simulink model "Foc"  (R2020b)
settings: Solver=FixedStepAuto  StartTime=0.0  StopTime=2  FixedStep=0.000001  RelTol=1e-3
libraries: powerlib x6, pid_lib x3, simulink x1
settings Model: Creator=Anson  LastModifiedBy=Anson

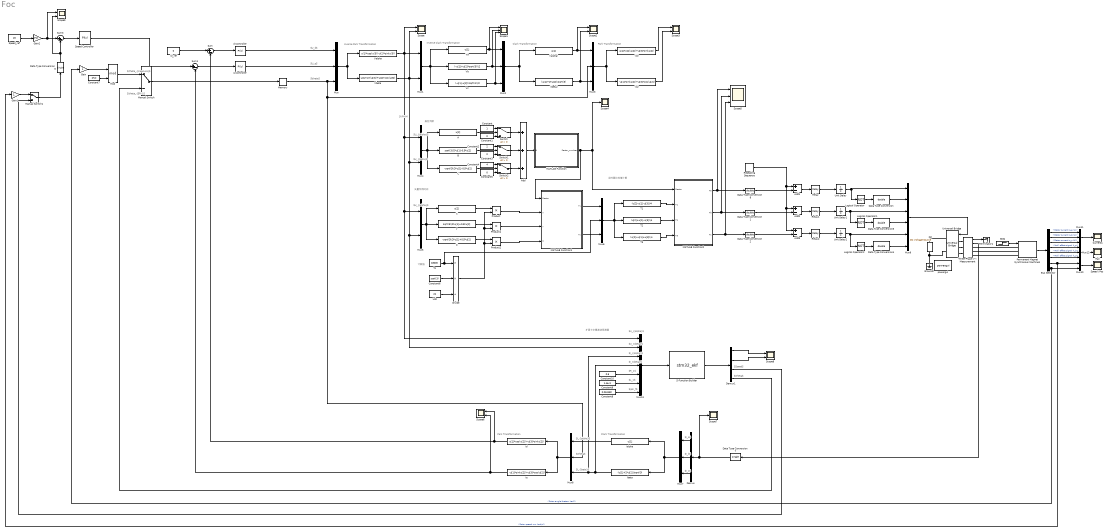
== system Foc ==
  note: $\theta$
  note: $U_q$
  note: $\theta$
  note: $\theta$
  note: $\theta_{EFK}$
  note: 扩展卡尔曼滤波观测器
  note: $I_a$
  note: $U_{\alpha}$
  note: 定时器比较值计算
  note: 矢量作用时间
  note: SVPWM
  note: 计数值
  note: Park Transformation
  note: Clark Transformation
  note: Inverse Clark Transformation
  note: Inverse Park Transformation
  note: 扇区判断
  note: Park Transformation
  note: Clark Transformation
  note: $U_{\beta}$
  note: $U_{\alpha}$
  note: $U_{\beta}$
  note: $I_b$
  note: $I_c$
  note: $U_{\alpha}$
  note: $I_{\alpha}$
  note: $I_{\beta}$
  note: $\psi_f$
  note: $L_s$
  note: $R_s$
  note: $\theta_{measure}$
  note: $U_d$
  note: $I_{\alpha}$
  note: $I_{\beta}$
  note: $Speed$
  (Ialpha) : Fcn  Expr=u[1]
  (Ibeta) : Fcn  Expr=(u[1]+2*u[2])/sqrt(3)
  (Id) : Fcn  Expr=u[1]*cos(u[2])+u[3]*sin(u[2])
  (Iq) : Fcn  Expr=-u[1]*sin(u[2])+u[3]*cos(u[2])
  A : Fcn  Expr=u[2]
  Add : Sum  Inputs=+++
  Add1 : Sum  Inputs=+-
  Add2 : Sum  Inputs=+-
  Add3 : Sum  Inputs=+-
  B : Fcn  Expr=sqrt(3)/2*u[1]-0.5*u[2]
  Bus Selector : BusSelector  OutputSignals=Stator current is_a (A),Stator current is_b (A),Stator current is_c (A),Hall effect signal h_a,Hall effect signal h_b,Hall effect signal h_c,Rotor speed wm (rad/s),Rotor angle thetam (rad)
  C : Fcn  Expr=-sqrt(3)/2*u[1]-0.5*u[2]
  Constant : Constant
  Constant1 : Constant  Value=0
  Constant10 : Constant  Value=0.6  OutDataTypeStr=single
  Constant2 : Constant  Value=2
  Constant3 : Constant  Value=0
  Constant4 : Constant  Value=4
  Constant5 : Constant  Value=0
  Constant6 : Constant  Value=sqrt(3)  OutDataTypeStr=single
  Constant7 : Constant  Value=2*pi  OutDataTypeStr=single
  Constant8 : Constant  Value=0.034182  OutDataTypeStr=single
  Constant9 : Constant  Value=1.4e-3  OutDataTypeStr=single
  Currents : Scope
  "DC " : powerlib/Electrical Sources/DC Voltage Source  Amplitude=24  Measurements=None
  Data Type Conversion{,1..4,8} (6 alike) : DataTypeConversion  OutDataTypeStr=double
  Data Type Conversion6 : DataTypeConversion  OutDataTypeStr=single
  Data Type Conversion7 : DataTypeConversion  OutDataTypeStr=single
  Demux : Demux  Outputs=3
  Demux1 : Demux
  Divide : Product  Inputs=**/
  Gain : Gain  OutDataTypeStr=single
  Gain1 : Gain  OutDataTypeStr=double
  Gain2 : Gain  Gain=2*pi  OutDataTypeStr=single
  Ground2 : powerlib/Elements/Ground  LConnTagsString=a
  Hall : Scope
  Ialpha : Fcn  Expr=u[1]
  Ibeta : Fcn  Expr=(u[1]+2*u[2])/sqrt(3)
  Id : Fcn  Expr=u[1]*cos(u[2])+u[3]*sin(u[2])
  Id_ref : Constant  Value=0  OutDataTypeStr=single
  Iq : Fcn  Expr=-u[1]*sin(u[2])+u[3]*cos(u[2])
  Logical Operator : Logic  Operator=NOT  AllPortsSameDT=off  OutDataTypeStr=boolean
  Logical Operator1 : Logic  Operator=NOT  AllPortsSameDT=off  OutDataTypeStr=boolean
  Logical Operator2 : Logic  Operator=NOT  AllPortsSameDT=off  OutDataTypeStr=boolean
  MATLAB Function : MATLAB Function  TreatAsAtomicUnit=on
  MATLAB Function1 : MATLAB Function  TreatAsAtomicUnit=on
  MATLAB Function2 : MATLAB Function  TreatAsAtomicUnit=on
  Manual Switch : ManualSwitch
  Manual Switch1 : ManualSwitch
  Memory : Memory
  Mod : Math  Operator=mod  SaturateOnIntegerOverflow=on
  Mux{,2..3,6..8,11..12} (8 alike) : Mux  Inputs=3
  Mux{1,4..5,10} (4 alike) : Mux  Inputs=2
  Mux13 : Mux  Inputs=7
  Mux9 : Mux  Inputs=6
  Permanent Magnet Synchronous Machine1 : powerlib/Machines/Permanent Magnet Synchronous Machine  NbPhases=3  FluxDistribution=Sinusoidal  RotorType=Round  MechanicalLoad=Torque Tm  PresetModel=No  ShowDetailedParameters=on  MeasurementBus=off  Resistance=0.6  Inductance=8.5e-3  dqInductances=[8.5e-3, 8.5e-3]  La=1.4e-3  MachineConstant=Flux linkage established by magnets (V.s)  Flux=0.034182  VoltageCst=6.1999  TorqueCst=0.051273  Flat=120  Mechanical=[1.1e-5,1e-4,1,0.02]  PolePairs=4  InitialConditions=[0,0, 0,0]  InitialConditions5ph=[0 0 0 0 0 0]  RefAngle=Aligned with phase A axis (original Park)  IterativeDiscreteModel=Trapezoidal non iterative  TsBlock=-1  TsPowergui=0
  Product : Product
  Product1 : Product
  Product2 : Product
  Relay : Relay  OffSwitchValue=-eps
  Relay1 : Relay  OffSwitchValue=-eps
  Relay2 : Relay  OffSwitchValue=-eps
  Repeating Sequence : simulink/Sources/Repeating Sequence  rep_seq_t=[0 0.0001 0.0002]  rep_seq_y=[0 9000 0]
  S-Function Builder : S-Function  InitFcn=try, set_param(gcb,'FunctionName','stm32_ekf'), end  FunctionName=stm32_ekf  SFunctionModules=stm32_ekf_wrapper  SFunctionDeploymentMode=off  EnableBusSupport=off  mask(S-Function Builder){}
      mask help: Simulink:masks:SFunctionBuilder_MD
      mask init:
      | val = [[.9  0.75 0.75 1 1 .9 .9 1]',[1 1 0.75 0.75 .9 .9 1 .9]'];try , sys = get_param(gcb,'SfunBuilderFcnName');if isempty(sys), sys = get_param(gcb,'FunctionName'); end,catch, sys = get_param(gcb,'FunctionName'); end
      settings: CopyFcn=set_param(gcbh,'LinkStatus','none')  PreSaveFcn=try, set_param(gcb,'FunctionName','stm32_ekf'), end  OpenFcn=sfunctionwizard(gcbh)
      mask Display: plot(val(:,1),val(:,2)),disp(sys),port_label('input',1,'u'),port_label('output',1,'y')
  Scope{,2..3,6,8..9} (6 alike) : Scope  NumInputPorts=2
  Scope1 : Scope  NumInputPorts=3
  Scope4 : Scope
  Scope5 : Scope  NumInputPorts=3
  Scope7 : Scope
  Speed / Pos : Scope
  Speed Controller : pid_lib/PID Controller  Controller=PI  Form=Ideal  TimeDomain=Discrete-time  UseExternalTs=off  SampleTime=-1  IntegratorMethod=Forward Euler  FilterMethod=Forward Euler  ControllerParametersSource=internal  P=0.005  I=6.0  D=0.0005  UseFilter=on  N=100  TunerSelectOption=Transfer Function Based (PID Tuner App)  InitialConditionSource=internal  InitialConditionForIntegrator=0  InitialConditionForFilter=0  DifferentiatorICPrevScaledInput=0  ExternalReset=none  TrackingMode=off  Kt=1  LimitOutput=on  SatLimitsSource=internal  UpperSaturationLimit=5.0  LowerSaturationLimit=-5.0  LinearizeAsGain=off  AntiWindupMode=back-calculation  Kb=0.015  PGainOutDataTypeStr=single  PProdOutDataTypeStr=single  POutMin=[]  POutMax=[]  IGainOutDataTypeStr=single  IProdOutDataTypeStr=single  IOutMin=[]  IOutMax=[]  DOutMin=[]  DOutMax=[]  NOutMin=[]  NOutMax=[]  SumOutDataTypeStr=single  SumOutMin=[]  SumOutMax=[]  SaturationOutDataTypeStr=single  SaturationOutMin=[]  SaturationOutMax=[]  PParamDataTypeStr=single  PParamMin=[]  PParamMax=[]  IParamDataTypeStr=single  IParamMin=[]  IParamMax=[]  DParamMin=[]  DParamMax=[]  NParamMin=[]  NParamMax=[]  KbParamDataTypeStr=single  KbParamMin=[]  KbParamMax=[]  KtParamMin=[]  KtParamMax=[]  KbOutDataTypeStr=single  KbOutMin=[]  KbOutMax=[]  KtOutMin=[]  KtOutMax=[]  IntegratorOutDataTypeStr=single  IntegratorOutMin=[]  IntegratorOutMax=[]  FilterOutMin=[]  FilterOutMax=[]  SumI1OutDataTypeStr=single  SumI1OutMin=[]  SumI1OutMax=[]  SumI2OutDataTypeStr=single  SumI2OutMin=[]  SumI2OutMax=[]  SumI3OutMin=[]  SumI3OutMax=[]  SumI4OutMin=[]  SumI4OutMax=[]  SumDOutMin=[]  SumDOutMax=[]  SumAccumDataTypeStr=single  SumI1AccumDataTypeStr=single  SumI2AccumDataTypeStr=single  DifferentiatorOutMin=[]  DifferentiatorOutMax=[]  FilterDiffOutCoefMin=[]  FilterDiffOutCoefMax=[]  ReciprocalOutMin=[]  ReciprocalOutMax=[]  SumDenOutMin=[]  SumDenOutMax=[]  SumNumOutMin=[]  SumNumOutMax=[]  DivideOutMin=[]  DivideOutMax=[]  UdiffTsProdOutMin=[]  UdiffTsProdOutMax=[]  NTsProdOutMin=[]  NTsProdOutMax=[]  UintegralTsProdOutMin=[]  UintegralTsProdOutMax=[]  UngainTsProdOutMin=[]  UngainTsProdOutMax=[]  IntegratorContinuousStateAttributes=''  IntegratorStateIdentifier=si  IntegratorStateMustResolveToSignalObject=off  IntegratorRTWStateStorageClass=Auto  FilterContinuousStateAttributes=''  FilterStateMustResolveToSignalObject=off  FilterRTWStateStorageClass=Auto  ParallelPVariant=Passthrough  IdealPVariant=InternalParameters  IVariant=InternalParameters  DVariant=Disabled  IntegratorVariant=Discrete  SatVariant=Enabled  AWVariant=BackCalculation  PCopyVariant=Disabled  TRVariant=Disabled  FdbkBlocksVariant=Forward  IdealPFdbkVariant=Disabled  SatFdbkVariant=Disabled  DerivativeFilterVariant=Disabled  NVariant=Disabled  NCopyVariant=Disabled_SignalSpec  FilterICVariant=Disabled  IntegratorICVariant=InternalICs  ExternalResetVariant=Disabled  TRSumVariant=Passthrough  SumFdbkVariant=Disabled  SumVariant=Sum_PI  TsampFilterVariant=InternalTs  TsampNgainVariant=Passthrough  TsampIntegralVariant=Passthrough  ExternalSaturationOutDataTypeStr=Inherit: Same as second input
  Speed_ref : Constant  Value=20  OutDataTypeStr=single
  Step : Step  Time=0  After=0  SampleTime=0
  Sum : Sum  Inputs=|+-
  Sum1 : Sum  Inputs=|+-
  Sum3 : Sum  Inputs=|+-  InputSameDT=on
  Switch : Switch  Criteria=u2 > Threshold
  Switch1 : Switch  Criteria=u2 > Threshold
  Switch2 : Switch  Criteria=u2 > Threshold
  T1 : Fcn  Expr=(u[2]-u[1]-u[3])/4
  T2 : Fcn  Expr=(u[2]+u[1]-u[3])/4
  T3 : Fcn  Expr=(u[2]+u[1]+u[3])/4
  Terminator1 : Terminator
  Three-Phase V-I Measurement : powerlib/Measurements/Three-Phase V-I Measurement  VoltageMeasurement=phase-to-ground  SetLabelV=off  LabelV=Vabc  Vpu=off  VpuLL=off  CurrentMeasurement=yes  SetLabelI=off  LabelI=Iabc  Ipu=off  Pbase=100e6  Vbase=500e3  OutputType=Complex  PhasorSimulation=off  PSBequivalent=0
  Ts : Constant  Value=18000  OutDataTypeStr=single
  Udc : Constant  Value=24  OutDataTypeStr=single
  Unit Delay : UnitDelay  SampleTime=-1  HasFrameUpgradeWarning=on
  Unit Delay1 : UnitDelay  SampleTime=-1  HasFrameUpgradeWarning=on
  Unit Delay2 : UnitDelay  SampleTime=-1  HasFrameUpgradeWarning=on
  Universal Bridge : powerlib/Power Electronics/Universal Bridge  Arms=3  SnubberResistance=1e5  SnubberCapacitance=inf  Device=IGBT / Diodes  Ron=1e-3  Lon=0  ForwardVoltages="[  0  0  ]"  ForwardVoltage=0  GTOparameters=[ 10e-6 , 20e-6 ]  IGBTparameters=[ 1e-6 , 2e-6 ]  Measurements=None  Measurements_2=None  converterType=Rectifier
  Va : Fcn  Expr=u[1]
  Valpha : Fcn  Expr=u(1)*cos(u(3))-u(2)*sin(u(3))
  Vb : Fcn  Expr=(-u[1]+u[2]*sqrt(3))/2
  Vbeta : Fcn  Expr=u[1]*sin(u[3])+u[2]*cos(u[3])
  Vc : Fcn  Expr=(-u[1]-u[2]*sqrt(3))/2
  X : Fcn  Expr=u[2]
  Y : Fcn  Expr=sqrt(3)/2*u[1]+0.5*u[2]
  Z : Fcn  Expr=-sqrt(3)/2*u[1]+0.5*u[2]
  d Controller : pid_lib/PID Controller  Controller=PI  Form=Parallel  TimeDomain=Discrete-time  UseExternalTs=off  SampleTime=-1  IntegratorMethod=Forward Euler  FilterMethod=Forward Euler  ControllerParametersSource=internal  P=2.199  I=1282.8  D=0.09  UseFilter=on  N=100  TunerSelectOption=Transfer Function Based (PID Tuner App)  InitialConditionSource=internal  InitialConditionForIntegrator=0  InitialConditionForFilter=0  DifferentiatorICPrevScaledInput=0  ExternalReset=none  TrackingMode=off  Kt=1  LimitOutput=on  SatLimitsSource=internal  UpperSaturationLimit=24  LowerSaturationLimit=-24  LinearizeAsGain=off  AntiWindupMode=back-calculation  Kb=15  PGainOutDataTypeStr=single  PProdOutDataTypeStr=single  POutMin=[]  POutMax=[]  IGainOutDataTypeStr=single  IProdOutDataTypeStr=single  IOutMin=[]  IOutMax=[]  DOutMin=[]  DOutMax=[]  NOutMin=[]  NOutMax=[]  SumOutDataTypeStr=single  SumOutMin=[]  SumOutMax=[]  SaturationOutDataTypeStr=single  SaturationOutMin=[]  SaturationOutMax=[]  PParamDataTypeStr=single  PParamMin=[]  PParamMax=[]  IParamDataTypeStr=single  IParamMin=[]  IParamMax=[]  DParamMin=[]  DParamMax=[]  NParamMin=[]  NParamMax=[]  KbParamDataTypeStr=single  KbParamMin=[]  KbParamMax=[]  KtParamMin=[]  KtParamMax=[]  KbOutDataTypeStr=single  KbOutMin=[]  KbOutMax=[]  KtOutMin=[]  KtOutMax=[]  IntegratorOutDataTypeStr=single  IntegratorOutMin=[]  IntegratorOutMax=[]  FilterOutMin=[]  FilterOutMax=[]  SumI1OutDataTypeStr=single  SumI1OutMin=[]  SumI1OutMax=[]  SumI2OutDataTypeStr=single  SumI2OutMin=[]  SumI2OutMax=[]  SumI3OutMin=[]  SumI3OutMax=[]  SumI4OutMin=[]  SumI4OutMax=[]  SumDOutMin=[]  SumDOutMax=[]  SumAccumDataTypeStr=single  SumI1AccumDataTypeStr=single  SumI2AccumDataTypeStr=single  DifferentiatorOutMin=[]  DifferentiatorOutMax=[]  FilterDiffOutCoefMin=[]  FilterDiffOutCoefMax=[]  ReciprocalOutMin=[]  ReciprocalOutMax=[]  SumDenOutMin=[]  SumDenOutMax=[]  SumNumOutMin=[]  SumNumOutMax=[]  DivideOutMin=[]  DivideOutMax=[]  UdiffTsProdOutMin=[]  UdiffTsProdOutMax=[]  NTsProdOutMin=[]  NTsProdOutMax=[]  UintegralTsProdOutMin=[]  UintegralTsProdOutMax=[]  UngainTsProdOutMin=[]  UngainTsProdOutMax=[]  IntegratorContinuousStateAttributes=''  IntegratorStateIdentifier=di  IntegratorStateMustResolveToSignalObject=off  IntegratorRTWStateStorageClass=Auto  FilterContinuousStateAttributes=''  FilterStateMustResolveToSignalObject=off  FilterRTWStateStorageClass=Auto  ParallelPVariant=InternalParameters  IdealPVariant=Disabled  IVariant=InternalParameters  DVariant=Disabled  IntegratorVariant=Discrete  SatVariant=Enabled  AWVariant=BackCalculation  PCopyVariant=Disabled  TRVariant=Disabled  FdbkBlocksVariant=Forward  IdealPFdbkVariant=Disabled  SatFdbkVariant=Disabled  DerivativeFilterVariant=Disabled  NVariant=Disabled  NCopyVariant=Disabled_SignalSpec  FilterICVariant=Disabled  IntegratorICVariant=InternalICs  ExternalResetVariant=Disabled  TRSumVariant=Passthrough  SumFdbkVariant=Disabled  SumVariant=Sum_PI  TsampFilterVariant=InternalTs  TsampNgainVariant=Passthrough  TsampIntegralVariant=Passthrough  ExternalSaturationOutDataTypeStr=Inherit: Same as second input
  powergui : powerlib/powergui  Priority=1  SimulationMode=Discrete  SampleTime=0.000001  frequency=60  Iterations=50  frequencyindice=0  Pbase=100e6  ErrMax=1e-4  UnitsV=kV  UnitsW=MW  buscounter=0  FunctionMessages=off  echomessages=off  EnableUseOfTLC=off  CurrentSourceSwitches=off  DisableSnubberDevices=off  DisableRonSwitches=off  DisableVfSwitches=off  DisplayEquations=off  AutomaticDiscreteSolvers=off  SolverType=Tustin/Backward Euler (TBE)  Interpol=off  ExternalGateDelay=off  methode=off  Ts=100  x0status=blocks  SPID=off  SwTol=0  HookPort=off  NonlinearTolerance=1e-4  nMaxIteration=100  ContinueOnMaxIteration=off  RestoreLinks=warning  ResistiveCurrentMeasurement=off  Frange=[0:2:500]  Ylog=off  Xlog=on  ShowGrid=off  save=off  variable=ZData  structure=0  ZoomFFT=off  StartTime=0.0  cycles=1  DisplayStyle=1  fundamental=60  FreqAxis=off  MaxFrequency=1000  frequencyindicesteady=1  RmsSteady=1  display=off
  q Controller : pid_lib/PID Controller  Controller=PI  Form=Parallel  TimeDomain=Discrete-time  UseExternalTs=off  SampleTime=-1  IntegratorMethod=Forward Euler  FilterMethod=Forward Euler  ControllerParametersSource=internal  P=2.199  I=1282.8  D=0.09  UseFilter=on  N=100  TunerSelectOption=Transfer Function Based (PID Tuner App)  InitialConditionSource=internal  InitialConditionForIntegrator=0  InitialConditionForFilter=0  DifferentiatorICPrevScaledInput=0  ExternalReset=none  TrackingMode=off  Kt=1  LimitOutput=on  SatLimitsSource=internal  UpperSaturationLimit=24  LowerSaturationLimit=-24  LinearizeAsGain=off  AntiWindupMode=back-calculation  Kb=15  PGainOutDataTypeStr=single  PProdOutDataTypeStr=single  POutMin=[]  POutMax=[]  IGainOutDataTypeStr=single  IProdOutDataTypeStr=single  IOutMin=[]  IOutMax=[]  DOutMin=[]  DOutMax=[]  NOutMin=[]  NOutMax=[]  SumOutDataTypeStr=single  SumOutMin=[]  SumOutMax=[]  SaturationOutDataTypeStr=single  SaturationOutMin=[]  SaturationOutMax=[]  PParamDataTypeStr=single  PParamMin=[]  PParamMax=[]  IParamDataTypeStr=single  IParamMin=[]  IParamMax=[]  DParamMin=[]  DParamMax=[]  NParamMin=[]  NParamMax=[]  KbParamDataTypeStr=single  KbParamMin=[]  KbParamMax=[]  KtParamMin=[]  KtParamMax=[]  KbOutDataTypeStr=single  KbOutMin=[]  KbOutMax=[]  KtOutMin=[]  KtOutMax=[]  IntegratorOutDataTypeStr=single  IntegratorOutMin=[]  IntegratorOutMax=[]  FilterOutMin=[]  FilterOutMax=[]  SumI1OutDataTypeStr=single  SumI1OutMin=[]  SumI1OutMax=[]  SumI2OutDataTypeStr=single  SumI2OutMin=[]  SumI2OutMax=[]  SumI3OutMin=[]  SumI3OutMax=[]  SumI4OutMin=[]  SumI4OutMax=[]  SumDOutMin=[]  SumDOutMax=[]  SumAccumDataTypeStr=single  SumI1AccumDataTypeStr=single  SumI2AccumDataTypeStr=single  DifferentiatorOutMin=[]  DifferentiatorOutMax=[]  FilterDiffOutCoefMin=[]  FilterDiffOutCoefMax=[]  ReciprocalOutMin=[]  ReciprocalOutMax=[]  SumDenOutMin=[]  SumDenOutMax=[]  SumNumOutMin=[]  SumNumOutMax=[]  DivideOutMin=[]  DivideOutMax=[]  UdiffTsProdOutMin=[]  UdiffTsProdOutMax=[]  NTsProdOutMin=[]  NTsProdOutMax=[]  UintegralTsProdOutMin=[]  UintegralTsProdOutMax=[]  UngainTsProdOutMin=[]  UngainTsProdOutMax=[]  IntegratorContinuousStateAttributes=''  IntegratorStateIdentifier=qi  IntegratorStateMustResolveToSignalObject=off  IntegratorRTWStateStorageClass=Auto  FilterContinuousStateAttributes=''  FilterStateMustResolveToSignalObject=off  FilterRTWStateStorageClass=Auto  ParallelPVariant=InternalParameters  IdealPVariant=Disabled  IVariant=InternalParameters  DVariant=Disabled  IntegratorVariant=Discrete  SatVariant=Enabled  AWVariant=BackCalculation  PCopyVariant=Disabled  TRVariant=Disabled  FdbkBlocksVariant=Forward  IdealPFdbkVariant=Disabled  SatFdbkVariant=Disabled  DerivativeFilterVariant=Disabled  NVariant=Disabled  NCopyVariant=Disabled_SignalSpec  FilterICVariant=Disabled  IntegratorICVariant=InternalICs  ExternalResetVariant=Disabled  TRSumVariant=Passthrough  SumFdbkVariant=Disabled  SumVariant=Sum_PI  TsampFilterVariant=InternalTs  TsampNgainVariant=Passthrough  TsampIntegralVariant=Passthrough  ExternalSaturationOutDataTypeStr=Inherit: Same as second input
  wires:
  (Id)/1 -> Scope3/1
  (Iq)/1 -> Scope3/2
  Mux3/1 -> (Iq)/1, (Id)/1
  (Ibeta)/1 -> Scope2/2, Mux3/3
  (Ialpha)/1 -> Scope2/1, Mux3/1
  Vc/1 -> Scope1/3, Mux2/3
  Mux2/1 -> (Ibeta)/1, (Ialpha)/1
  Vb/1 -> Scope1/2, Mux2/2
  Valpha/1 -> Mux13/1, Mux5/1, Mux4/1, Scope/1, Mux1/1
  Mux1/1 -> Va/1, Vc/1, Vb/1
  Va/1 -> Scope1/1, Mux2/1
  Vbeta/1 -> Mux4/2, Mux5/2, Mux13/2, Scope/2, Mux1/2
  Mux/1 -> Valpha/1, Vbeta/1
  Mux4/1 -> A/1, C/1, B/1
  A/1 -> Switch/2
  B/1 -> Switch1/2
  C/1 -> Switch2/2
  Constant/1 -> Switch/1
  Constant1/1 -> Switch/3
  Constant2/1 -> Switch1/1
  Constant3/1 -> Switch1/3
  Constant4/1 -> Switch2/1
  Constant5/1 -> Switch2/3
  Switch1/1 -> Add/2
  Switch2/1 -> Add/3
  Switch/1 -> Add/1
  Add/1 -> MATLAB Function/1(N)
  MATLAB Function/1(Sector_number) -> MATLAB Function2/1(Sector), Scope4/1, MATLAB Function1/1(Sector)
  Mux5/1 -> X/1, Z/1, Y/1
  X/1 -> Product/1
  Y/1 -> Product1/1
  Z/1 -> Product2/1
  Divide/1 -> Product2/2, Product1/2, Product/2
  Product/1 -> MATLAB Function1/2(X)
  Product1/1 -> MATLAB Function1/3(Y)
  Product2/1 -> MATLAB Function1/4(Z)
  MATLAB Function1/1(Tx) -> Mux6/1
  MATLAB Function1/2(Ty) -> Mux6/3
  Mux6/1 -> T3/1, T1/1, T2/1
  T3/1 -> MATLAB Function2/4(T3)
  T2/1 -> MATLAB Function2/3(T2)
  T1/1 -> MATLAB Function2/2(T1)
  MATLAB Function2/2(Tb) -> Data Type Conversion1/1, Scope5/2
  MATLAB Function2/3(Tc) -> Data Type Conversion2/1, Scope5/3
  Mux8/1 -> Iq/1, Id/1
  Mux7/1 -> Ibeta/1, Ialpha/1
  Ibeta/1 -> Mux13/4, Mux13/3, Mux8/3
  Ialpha/1 -> Mux8/1
  MATLAB Function2/1(Ta) -> Data Type Conversion8/1, Scope5/1
  Data Type Conversion3/1 -> Mux9/4
  Add1/1 -> Relay/1
  Relay/1 -> Unit Delay/1
  Repeating Sequence/1 -> Add3/1, Add2/1, Add1/1
  Unit Delay2/1 -> Mux9/5, Logical Operator2/1
  Add3/1 -> Relay2/1
  Logical Operator2/1 -> Data Type Conversion4/1
  Relay1/1 -> Unit Delay1/1
  Add2/1 -> Relay1/1
  Unit Delay/1 -> Logical Operator/1, Mux9/1
  Logical Operator1/1 -> Data Type Conversion3/1
  Mux9/1 -> Universal Bridge/1
  Data Type Conversion4/1 -> Mux9/6
  Data Type Conversion/1 -> Mux9/2
  Data Type Conversion2/1 -> Add3/2
  Unit Delay1/1 -> Logical Operator1/1, Mux9/3
  Relay2/1 -> Unit Delay2/1
  Data Type Conversion8/1 -> Add1/2
  Data Type Conversion1/1 -> Add2/2
  Logical Operator/1 -> Data Type Conversion/1
  Step/1 -> Permanent Magnet Synchronous Machine1/1
  Demux/1 -> Mux7/1
  Demux/2 -> Mux7/2
  Demux/3 -> Mux7/3
  Three-Phase V-I Measurement/2 -> Data Type Conversion7/1
  Three-Phase V-I Measurement/1 -> Terminator1/1
  d Controller/1 -> Mux/1
  Speed Controller/1 -> Sum1/1
  Id/1 -> Sum/2, Scope6/1
  Iq/1 -> Sum1/2, Scope6/2
  Bus Selector/5 -> Mux12/2  "<Hall effect signal h_b>"
  Bus Selector/2 -> Mux11/2  "<Stator current is_b (A)>"
  Bus Selector/3 -> Mux11/3  "<Stator current is_c (A)>"
  Bus Selector/1 -> Mux11/1  "<Stator current is_a (A)>"
  Bus Selector/8 -> Gain/1, Mux10/2  "<Rotor angle thetam (rad)>"
  Bus Selector/6 -> Mux12/3  "<Hall effect signal h_c>"
  Permanent Magnet Synchronous Machine1/1 -> Bus Selector/1
  Bus Selector/4 -> Mux12/1  "<Hall effect signal h_a>"
  Mux10/1 -> Speed / Pos/1
  Mux11/1 -> Currents/1
  Bus Selector/7 -> Gain1/1, Mux10/1  "<Rotor speed wm (rad/s)>"
  Mux12/1 -> Hall/1
  Constant7/1 -> Mod/2
  Gain/1 -> Mod/1
  Mux13/1 -> S-Function Builder/1
  S-Function Builder/1 -> Demux1/1
  Mod/1 -> Manual Switch/1
  Demux1/4 -> Manual Switch/2
  Demux1/1 -> Scope8/1
  Demux1/2 -> Scope8/2
  Demux1/3 -> Manual Switch1/2
  Sum3/1 -> Speed Controller/1
  Manual Switch1/1 -> Data Type Conversion6/1
  Gain2/1 -> Scope9/1, Sum3/1
  Gain1/1 -> Manual Switch1/1
  Manual Switch/1 -> Memory/1
  Constant8/1 -> Mux13/7
  Constant9/1 -> Mux13/6
  Constant10/1 -> Mux13/5
  Ts/1 -> Mux6/2, Divide/1
  Constant6/1 -> Divide/2
  Udc/1 -> Divide/3
  Id_ref/1 -> Sum/1
  Data Type Conversion7/1 -> Scope7/1, Demux/1
  Speed_ref/1 -> Gain2/1
  Data Type Conversion6/1 -> Scope9/2, Sum3/2
  Sum/1 -> d Controller/1
  Sum1/1 -> q Controller/1
  q Controller/1 -> Mux/2
  Memory/1 -> Mux3/2, Mux8/2, Mux/3
  connections:
  Ground2/LConn1 -- Universal Bridge/RConn2 -- "DC "/LConn1
  Universal Bridge/LConn1 -- Three-Phase V-I Measurement/LConn1
  Permanent Magnet Synchronous Machine1/LConn3 -- Three-Phase V-I Measurement/RConn3
  Permanent Magnet Synchronous Machine1/LConn2 -- Three-Phase V-I Measurement/RConn2
  Permanent Magnet Synchronous Machine1/LConn1 -- Three-Phase V-I Measurement/RConn1
  "DC "/RConn1 -- Universal Bridge/RConn1
  Universal Bridge/LConn3 -- Three-Phase V-I Measurement/LConn3
  Universal Bridge/LConn2 -- Three-Phase V-I Measurement/LConn2

== matlab function Foc/MATLAB Function1 ==
  data: Sector input; X input; Tx output; Y input; Z input; Ty output
function [Tx, Ty] = fcn(Sector, X, Y, Z)
switch(Sector)
    case 1
         Tx = -Z;
         Ty = X;
    case 2
        Tx = Z;
        Ty = Y;
    case 3
        Tx = X;
        Ty = -Y;
    case 4
        Tx = -X;
        Ty = Z;
    case 5
        Tx = -Y;
        Ty = -Z;
    otherwise 
        Tx = Y;
        Ty = -X;
end

== matlab function Foc/MATLAB Function ==
  data: N input; Sector_number output
function Sector_number = fcn(N)
if N == 3
    Sector_number = 1;
elseif N == 1
    Sector_number = 2;
elseif N == 5
    Sector_number = 3;
elseif N == 4
    Sector_number = 4;
elseif N == 6
    Sector_number = 5;
else
    Sector_number = 6;
end

== matlab function Foc/MATLAB Function2 ==
  data: Sector input; T1 input; Ta output; T2 input; T3 input; Tb output; Tc output
function [Ta, Tb, Tc] = fcn(Sector, T1, T2, T3)
switch(Sector)
    case 1
        Ta = T1;
        Tb = T2;
        Tc = T3;
    case 2
        Ta = T2;
        Tb = T1;
        Tc = T3;
    case 3
        Ta = T3;
        Tb = T1;
        Tc = T2;
    case 4
        Ta = T3;
        Tb = T2;
        Tc = T1;
    case 5
        Ta = T2;
        Tb = T3;
        Tc = T1;
    otherwise 
        Ta = T1;
        Tb = T3;
        Tc = T2;
end
